simulink model "mcdc_test"  (R2017b)
settings: Solver=FixedStepDiscrete  StartTime=0.0  StopTime=10.0  FixedStep=0.200000  RelTol=1e-3  EnableMultiTasking=on
settings Model: Creator=arnaud  LastModifiedBy=hbourbou
settings DataIOCC: LimitDataPoints=on  SaveFormat=Structure  SignalLoggingSaveFormat=ModelDataLogs
settings OptimizationCC: ExpressionDepthLimit=2147483647  LifeSpan=inf
settings DebuggingCC: AlgebraicLoopMsg=error  ArtificialAlgebraicLoopMsg=error  UnderspecifiedInitializationDetection=Classic  MergeDetectMultiDrivingBlocksExec=none  SolverPrmCheckMsg=warning  SingleTaskRateTransMsg=error  FcnCallInpInsideContextMsg=warning  StateNameClashWarn=warning  SFUnexpectedBacktrackingDiag=warning  SFNoUnconditionalDefaultTransitionDiag=warning  SFExecutionAtInitializationDiag=none
settings HardwareCC: ProdBitPerPointer=32  ProdBitPerSizeT=32  ProdBitPerPtrDiffT=32  ProdLargestAtomicFloat=None  ProdIntDivRoundTo=Undefined  ProdEndianess=Unspecified  ProdWordSize=32  ProdHWDeviceType=32-bit Generic
settings ModelReferenceCC: PropagateSignalLabelsOutOfModel=off
settings CodeAppCC: StateflowObjectComments=on
settings GRTTargetCC: TargetLangStandard=C89/C90 (ANSI)  GeneratePreprocessorConditionals=Disable all  CombineOutputUpdateFcns=off  GRTInterface=on
settings ConfigComp: CovMetricSettings=dw  CovHtmlReporting=on  CovSaveCumulativeToWorkspaceVar=on  CovSaveSingleToWorkspaceVar=on  CovExternalEMLEnable=off  CovSFcnEnable=off

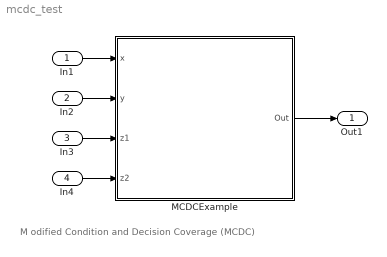
== system mcdc_test ==
  note: M odified Condition and Decision Coverage (MCDC)
  In1 : Inport  OutDataTypeStr=int32
  In2 : Inport  Port=2  OutDataTypeStr=int32
  In3 : Inport  Port=3  OutDataTypeStr=int32
  In4 : Inport  Port=4  OutDataTypeStr=int32
  MCDCExample : Subsystem  TreatAsAtomicUnit=on
  Out1 : Outport
  wires:
  MCDCExample/1(Out) -> Out1/1
  In1/1 -> MCDCExample/1(x)
  In2/1 -> MCDCExample/2(y)
  In3/1 -> MCDCExample/3(z1)
  In4/1 -> MCDCExample/4(z2)

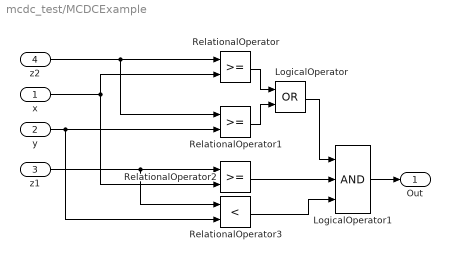
== system mcdc_test/MCDCExample ==
  x : Inport
  y : Inport  Port=2
  z1 : Inport  Port=3
  z2 : Inport  Port=4
  LogicalOperator : Logic  Operator=OR  AllPortsSameDT=off  OutDataTypeStr=boolean
  LogicalOperator1 : Logic  Inputs=3  AllPortsSameDT=off  OutDataTypeStr=boolean
  RelationalOperator : RelationalOperator  OutDataTypeStr=boolean  RndMeth=Nearest
  RelationalOperator1 : RelationalOperator  OutDataTypeStr=boolean  RndMeth=Nearest
  RelationalOperator2 : RelationalOperator  OutDataTypeStr=boolean  RndMeth=Nearest
  RelationalOperator3 : RelationalOperator  Operator=<  OutDataTypeStr=boolean  RndMeth=Nearest
  Out : Outport
  wires:
  RelationalOperator/1 -> LogicalOperator/1
  RelationalOperator1/1 -> LogicalOperator/2
  LogicalOperator/1 -> LogicalOperator1/1
  z2/1 -> RelationalOperator/1, RelationalOperator1/1
  LogicalOperator1/1 -> Out/1
  RelationalOperator2/1 -> LogicalOperator1/2
  RelationalOperator3/1 -> LogicalOperator1/3
  z1/1 -> RelationalOperator3/1, RelationalOperator2/1
  y/1 -> RelationalOperator3/2, RelationalOperator1/2
  x/1 -> RelationalOperator/2, RelationalOperator2/2
